simulink library "jud"  (Simulink 8.2)
settings: Solver=ode45  StartTime=0.0  StopTime=10.0  RelTol=1e-3
undefined symbols (not defined in the file or in its folder): ENUM_EPSADASABREASON_GEAR_POSITION_ERROR, ENUM_EPSADASABREASON_THERMAL_ERROR, ENUM_EPSADASABREASON_VEHICLE_SPEED_ERROR, ENUM_EPSLFCSTATUS_NOTAVAIL_PERM, ENUM_EPSLFCSTATUS_NOTAVAIL_TEMP, ENUM_EPSLFCSTATUS_OFF, ENUM_EPSLFCSTATUS_READY, ENUM_EPSLFCSTATUS_TRANSITION, ENUM_EPSLKASTATUS_NOTAVAIL_PERM, ENUM_EPSLKASTATUS_NOTAVAIL_TEMP, ENUM_EPSLKASTATUS_OFF, ENUM_EPSLKASTATUS_READY, ENUM_HMISTATE_ACTIVE, ENUM_KEYSWITCH_ON, ENUM_LFCSTATE_AUTOSTEERING, ENUM_LFCSTATE_STANDBY, ENUM_SENSORSTATE_NORMAL, FALSE, KAPP_VehicleWidth_m, KJUD_EPSLimition_kph, KJUD_EPSLimitionHysis_kph, KJUD_LFC4StandbyDelay_s, KJUD_SoftenTimerThr_s, TRUE, VJUD_LFCOffCount4LKAStandby_s, VJUD_LKAReActingDelay_s, VJUD_TLCTriggerReActingDelay_s
libraries: hcu_lib x12, simulink x10, jcc x1, jcw x1, jeb x1
(part 3 of 3)

== system jud/JUD/jud/JLKA/jka/LKA_LeftOperationalRecover_Conditions ==
  VIFO_LeftLaneCrossing_flg : Inport
  VPER_LaneC0L_m : Inport  Port=2
  VPER_LaneC1L_rad : Inport  Port=3
  Add1 : Sum  Inputs=+-
  C0L4Disabled : Constant  Value=-0.2
  C1L4Disabled : Constant  Value=-0.01
  C1L_Pos_sec : Constant  Value=0.5
  Compare To Zero : simulink/Logic and Bit Operations/Compare To Zero  relop=>=  OutDataTypeStr=boolean
  Gain2 : Gain  Gain=0.5
  "KAPP_VehicleWidth_m " : Constant  Value=KAPP_VehicleWidth_m
  Logical Operator4 : Logic  Inputs=3  AllPortsSameDT=off  OutDataTypeStr=boolean
  Logical Operator5 : Logic  Operator=OR  AllPortsSameDT=off  OutDataTypeStr=boolean
  Relational Operator4 : RelationalOperator  OutDataTypeStr=boolean
  Relational Operator5 : RelationalOperator  OutDataTypeStr=boolean
  Relational Operator6 : RelationalOperator  OutDataTypeStr=boolean
  Timer : hcu_lib/Timer  SystemSampleTime=-1
  VJUD_LKALeftOperationalRecover_flg : Outport
  wires:
  "KAPP_VehicleWidth_m "/1 -> Gain2/1
  Gain2/1 -> Add1/2
  VPER_LaneC0L_m/1 -> Add1/1
  VPER_LaneC1L_rad/1 -> Compare To Zero/1, Relational Operator4/1
  C1L4Disabled/1 -> Relational Operator4/2
  C0L4Disabled/1 -> Relational Operator5/2
  Add1/1 -> Relational Operator5/1  "VJUD_LaneC0L2Veh_m"
  Compare To Zero/1 -> Timer/Enable
  Timer/1 -> Relational Operator6/1
  C1L_Pos_sec/1 -> Relational Operator6/2
  Relational Operator4/1 -> Logical Operator4/1
  Relational Operator6/1 -> Logical Operator4/2
  Relational Operator5/1 -> Logical Operator4/3
  Logical Operator5/1 -> VJUD_LKALeftOperationalRecover_flg/1  "VJUD_LKALeftOperationalRecover_flg"
  Logical Operator4/1 -> Logical Operator5/1
  VIFO_LeftLaneCrossing_flg/1 -> Logical Operator5/2

== system jud/JUD/jud/JLKA/jka/LKA_NoADASFailre_Conditions ==
  VDHP_DisableLKA_flg : Inport
  Logical Operator1 : Logic  Operator=NOT  AllPortsSameDT=off  OutDataTypeStr=boolean
  VJUD_LKANoADASFailure_flg : Outport
  wires:
  Logical Operator1/1 -> VJUD_LKANoADASFailure_flg/1  "VJUD_LKANoADASFailure_flg"
  VDHP_DisableLKA_flg/1 -> Logical Operator1/1

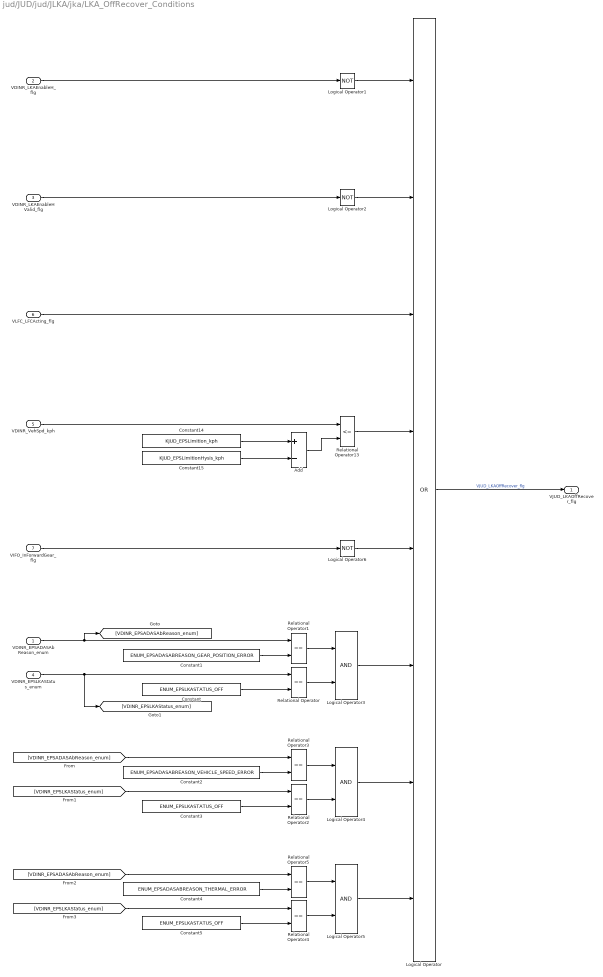
== system jud/JUD/jud/JLKA/jka/LKA_OffRecover_Conditions ==
  VDINR_EPSADASAbReason_enum : Inport
  VDINR_LKAEnableH_flg : Inport  Port=2
  VDINR_LKAEnableHValid_flg : Inport  Port=3
  VDINR_EPSLKAStatus_enum : Inport  Port=4
  VDINR_VehSpd_kph : Inport  Port=5
  VLFC_LFCActing_flg : Inport  Port=6
  VIFO_InForwardGear_flg : Inport  Port=7
  Add : Sum  Inputs=+-
  Constant : Constant  Value=ENUM_EPSLKASTATUS_OFF
  Constant1 : Constant  Value=ENUM_EPSADASABREASON_GEAR_POSITION_ERROR
  Constant14 : Constant  Value=KJUD_EPSLimition_kph
  Constant15 : Constant  Value=KJUD_EPSLimitionHysis_kph
  Constant2 : Constant  Value=ENUM_EPSADASABREASON_VEHICLE_SPEED_ERROR
  Constant3 : Constant  Value=ENUM_EPSLKASTATUS_OFF
  Constant4 : Constant  Value=ENUM_EPSADASABREASON_THERMAL_ERROR
  Constant5 : Constant  Value=ENUM_EPSLKASTATUS_OFF
  Logical Operator : Logic  Operator=OR  Inputs=8  AllPortsSameDT=off  OutDataTypeStr=boolean
  Logical Operator1 : Logic  Operator=NOT  AllPortsSameDT=off  OutDataTypeStr=boolean
  Logical Operator2 : Logic  Operator=NOT  AllPortsSameDT=off  OutDataTypeStr=boolean
  Logical Operator3 : Logic  AllPortsSameDT=off  OutDataTypeStr=boolean
  Logical Operator4 : Logic  AllPortsSameDT=off  OutDataTypeStr=boolean
  Logical Operator5 : Logic  AllPortsSameDT=off  OutDataTypeStr=boolean
  Logical Operator6 : Logic  Operator=NOT  AllPortsSameDT=off  OutDataTypeStr=boolean
  Relational Operator{,1..5} (6 alike) : RelationalOperator  Operator===  OutDataTypeStr=boolean
  Relational Operator13 : RelationalOperator  Operator=<=  OutDataTypeStr=boolean
  VJUD_LKAOffRecover_flg : Outport
  wires:
  Logical Operator/1 -> VJUD_LKAOffRecover_flg/1  "VJUD_LKAOffRecover_flg"
  Constant/1 -> Relational Operator/2
  VDINR_EPSLKAStatus_enum/1 -> [VDINR_EPSLKAStatus_enum], Relational Operator/1
  Relational Operator/1 -> Logical Operator3/2
  VDINR_EPSADASAbReason_enum/1 -> [VDINR_EPSADASAbReason_enum], Relational Operator1/1
  Constant1/1 -> Relational Operator1/2
  Relational Operator1/1 -> Logical Operator3/1
  [VDINR_EPSLKAStatus_enum] -> Relational Operator2/1
  Relational Operator2/1 -> Logical Operator4/2
  Constant2/1 -> Relational Operator3/2
  Relational Operator3/1 -> Logical Operator4/1
  [VDINR_EPSADASAbReason_enum] -> Relational Operator3/1
  Constant3/1 -> Relational Operator2/2
  [VDINR_EPSLKAStatus_enum] -> Relational Operator4/1
  Relational Operator4/1 -> Logical Operator5/2
  Constant4/1 -> Relational Operator5/2
  Relational Operator5/1 -> Logical Operator5/1
  [VDINR_EPSADASAbReason_enum] -> Relational Operator5/1
  Constant5/1 -> Relational Operator4/2
  VDINR_LKAEnableH_flg/1 -> Logical Operator1/1
  VDINR_LKAEnableHValid_flg/1 -> Logical Operator2/1
  VDINR_VehSpd_kph/1 -> Relational Operator13/1
  Constant14/1 -> Add/1
  Constant15/1 -> Add/2
  Add/1 -> Relational Operator13/2
  Logical Operator1/1 -> Logical Operator/1
  Logical Operator2/1 -> Logical Operator/2
  VLFC_LFCActing_flg/1 -> Logical Operator/3
  Relational Operator13/1 -> Logical Operator/4
  Logical Operator6/1 -> Logical Operator/5
  VIFO_InForwardGear_flg/1 -> Logical Operator6/1
  Logical Operator3/1 -> Logical Operator/6
  Logical Operator4/1 -> Logical Operator/7
  Logical Operator5/1 -> Logical Operator/8

== system jud/JUD/jud/JLKA/jka/LKA_Operational_Conditions ==
  VIFO_LeftLaneAvail_flg : Inport
  VIFO_RightLaneAvail_flg : Inport  Port=2
  VIFO_DriverTurningSignal_flg : Inport  Port=3
  VIFO_LKASpdInRange_flg : Inport  Port=4
  VIFO_Curvature4Disable_flg : Inport  Port=5
  VFCW_FCWStateHMI_enum : Inport  Port=6
  VAEB_AEBStateHMI_enum : Inport  Port=7
  Constant1 : Constant  Value=ENUM_HMISTATE_ACTIVE
  Constant2 : Constant  Value=ENUM_HMISTATE_ACTIVE
  Logical Operator : Logic  Inputs=6  AllPortsSameDT=off  OutDataTypeStr=boolean
  Logical Operator1 : Logic  Operator=OR  AllPortsSameDT=off  OutDataTypeStr=boolean
  Logical Operator2 : Logic  Operator=NOT  AllPortsSameDT=off  OutDataTypeStr=boolean
  Logical Operator3 : Logic  Operator=NOT  AllPortsSameDT=off  OutDataTypeStr=boolean
  Relational Operator2 : RelationalOperator  Operator=~=  OutDataTypeStr=boolean
  Relational Operator3 : RelationalOperator  Operator=~=  OutDataTypeStr=boolean
  VJUD_LKAOperationalReq_flg : Outport
  wires:
  Logical Operator/1 -> VJUD_LKAOperationalReq_flg/1  "VJUD_LKAOperationalReq_flg"
  VIFO_LeftLaneAvail_flg/1 -> Logical Operator1/1
  VIFO_RightLaneAvail_flg/1 -> Logical Operator1/2
  Logical Operator1/1 -> Logical Operator/1
  VIFO_DriverTurningSignal_flg/1 -> Logical Operator2/1
  VIFO_Curvature4Disable_flg/1 -> Logical Operator3/1
  VIFO_LKASpdInRange_flg/1 -> Logical Operator/2
  Logical Operator3/1 -> Logical Operator/3
  Logical Operator2/1 -> Logical Operator/4
  VFCW_FCWStateHMI_enum/1 -> Relational Operator2/1
  VAEB_AEBStateHMI_enum/1 -> Relational Operator3/1
  Constant1/1 -> Relational Operator2/2
  Constant2/1 -> Relational Operator3/2
  Relational Operator3/1 -> Logical Operator/6
  Relational Operator2/1 -> Logical Operator/5

== system jud/JUD/jud/JLKA/jka/LKA_RightAction_Conditions ==
  VDINR_EPSLKAStatus_enum : Inport
  VIFO_EPSStateChgAllow_flg : Inport  Port=2
  VIFO_TLCLTrigger_flg : Inport  Port=3
  VIFO_TLCRTrigger_flg : Inport  Port=4
  VLKA_LKAActing_flg : Inport  Port=5
  Constant1 : Constant  Value=ENUM_EPSLKASTATUS_READY
  Logical Operator : Logic  Operator=NOT  AllPortsSameDT=off  OutDataTypeStr=boolean
  Logical Operator3 : Logic  Inputs=5  AllPortsSameDT=off  OutDataTypeStr=boolean
  Logical Operator4 : Logic  Operator=NOT  AllPortsSameDT=off  OutDataTypeStr=boolean
  Relational Operator1 : RelationalOperator  RequirementInfo={} %GIDa_5d33ed69_386a_439d_af12_c65accea3bf3  Operator===  OutDataTypeStr=boolean
  Relational Operator2 : RelationalOperator  OutDataTypeStr=boolean
  Relational Operator3 : RelationalOperator  OutDataTypeStr=boolean
  Timer : hcu_lib/Timer  SystemSampleTime=-1
  Timer1 : hcu_lib/Timer  SystemSampleTime=-1
  VJUD_LKAReActingDelay_s : Constant  Value=VJUD_LKAReActingDelay_s
  VJUD_TLCTriggerReActingDelay_s : Constant  Value=VJUD_TLCTriggerReActingDelay_s
  VJUD_LKARightActionReq_flg : Outport
  wires:
  VIFO_TLCLTrigger_flg/1 -> Logical Operator/1
  Constant1/1 -> Relational Operator1/2
  VDINR_EPSLKAStatus_enum/1 -> Relational Operator1/1
  Logical Operator3/1 -> VJUD_LKARightActionReq_flg/1  "VJUD_LKARightActionReq_flg"
  VIFO_TLCRTrigger_flg/1 -> Logical Operator3/1
  Timer/1 -> Relational Operator2/1
  VJUD_LKAReActingDelay_s/1 -> Relational Operator2/2
  Logical Operator4/1 -> Timer/Enable
  VIFO_EPSStateChgAllow_flg/1 -> Logical Operator3/5
  Relational Operator1/1 -> Logical Operator3/4
  VLKA_LKAActing_flg/1 -> Logical Operator4/1
  Relational Operator2/1 -> Logical Operator3/2
  VJUD_TLCTriggerReActingDelay_s/1 -> Relational Operator3/2
  Relational Operator3/1 -> Logical Operator3/3
  Logical Operator/1 -> Timer1/Enable
  Timer1/1 -> Relational Operator3/1

== system jud/JUD/jud/JLKA/jka/LKA_RightOperationalRecover_Conditions ==
  VIFO_RightLaneCrossing_flg : Inport
  VPER_LaneC0R_m : Inport  Port=2
  VPER_LaneC1R_rad : Inport  Port=3
  Add1 : Sum
  C0R4Disabled : Constant  Value=0.2
  C1R4Disabled : Constant  Value=0.01
  C1R_nec_sec : Constant  Value=0.5
  Compare To Zero : simulink/Logic and Bit Operations/Compare To Zero  relop=<=  OutDataTypeStr=boolean
  Gain2 : Gain  Gain=0.5
  "KAPP_VehicleWidth_m " : Constant  Value=KAPP_VehicleWidth_m
  Logical Operator2 : Logic  Operator=OR  AllPortsSameDT=off  OutDataTypeStr=boolean
  Logical Operator4 : Logic  Inputs=3  AllPortsSameDT=off  OutDataTypeStr=boolean
  Relational Operator2 : RelationalOperator  Operator=<=  OutDataTypeStr=boolean
  Relational Operator3 : RelationalOperator  Operator=<=  OutDataTypeStr=boolean
  Relational Operator6 : RelationalOperator  OutDataTypeStr=boolean
  Timer : hcu_lib/Timer  SystemSampleTime=-1
  VJUD_LKARightOperationalRecover_flg : Outport
  wires:
  Add1/1 -> Relational Operator3/1  "VJUD_LaneC0R2Veh_m"
  "KAPP_VehicleWidth_m "/1 -> Gain2/1
  Gain2/1 -> Add1/2
  VPER_LaneC0R_m/1 -> Add1/1
  C1R4Disabled/1 -> Relational Operator2/2
  VPER_LaneC1R_rad/1 -> Compare To Zero/1, Relational Operator2/1
  Compare To Zero/1 -> Timer/Enable
  Timer/1 -> Relational Operator6/1
  C1R_nec_sec/1 -> Relational Operator6/2
  C0R4Disabled/1 -> Relational Operator3/2
  Relational Operator2/1 -> Logical Operator4/1
  Relational Operator6/1 -> Logical Operator4/2
  Logical Operator2/1 -> VJUD_LKARightOperationalRecover_flg/1  "VJUD_LKARightOperationalRecover_flg"
  Logical Operator4/1 -> Logical Operator2/1
  VIFO_RightLaneCrossing_flg/1 -> Logical Operator2/2
  Relational Operator3/1 -> Logical Operator4/3

== system jud/JUD/jud/JLKA/jka/LKA_StandbyRecover_Conditions ==
  VIFO_LaneNotAvail_flg : Inport
  VIFO_DriverTurningSignal_flg : Inport  Port=2
  VIFO_LKASpdInRange_flg : Inport  Port=3
  VIFO_Curvature4Disable_flg : Inport  Port=4
  VIFO_DriverStrFight_flg : Inport  Port=5
  VFCW_FCWStateHMI_enum : Inport  Port=6
  VAEB_AEBStateHMI_enum : Inport  Port=7
  Constant1 : Constant  Value=ENUM_HMISTATE_ACTIVE
  Constant2 : Constant  Value=ENUM_HMISTATE_ACTIVE
  Logical Operator : Logic  Operator=OR  Inputs=7  AllPortsSameDT=off  OutDataTypeStr=boolean
  Logical Operator1 : Logic  Operator=NOT  AllPortsSameDT=off  OutDataTypeStr=boolean
  Relational Operator2 : RelationalOperator  Operator===  OutDataTypeStr=boolean
  Relational Operator3 : RelationalOperator  Operator===  OutDataTypeStr=boolean
  VJUD_LKAStandbyRecover_flg : Outport
  wires:
  Logical Operator/1 -> VJUD_LKAStandbyRecover_flg/1  "VJUD_LKAStandbyRecover_flg"
  VIFO_DriverTurningSignal_flg/1 -> Logical Operator/2
  VIFO_LaneNotAvail_flg/1 -> Logical Operator/1
  VIFO_Curvature4Disable_flg/1 -> Logical Operator/4
  VIFO_DriverStrFight_flg/1 -> Logical Operator/5
  VIFO_LKASpdInRange_flg/1 -> Logical Operator1/1
  VFCW_FCWStateHMI_enum/1 -> Relational Operator2/1
  VAEB_AEBStateHMI_enum/1 -> Relational Operator3/1
  Constant1/1 -> Relational Operator2/2
  Constant2/1 -> Relational Operator3/2
  Relational Operator2/1 -> Logical Operator/6
  Relational Operator3/1 -> Logical Operator/7
  Logical Operator1/1 -> Logical Operator/3

== system jud/JUD/jud/JLKA/jka/LKA_TempFailureRecover_Conditions ==
  VDINR_EPSLKAStatus_enum : Inport
  VDHP_DisableADASFun_flg : Inport  Port=2
  Constant : Constant  Value=ENUM_EPSLKASTATUS_OFF
  Constant1 : Constant  Value=ENUM_EPSLKASTATUS_NOTAVAIL_PERM
  Logical Operator : Logic  Operator=OR  Inputs=3  AllPortsSameDT=off  OutDataTypeStr=boolean
  Relational Operator : RelationalOperator  Operator===  OutDataTypeStr=boolean
  Relational Operator2 : RelationalOperator  Operator===  OutDataTypeStr=boolean
  VJUD_LKATempFailureRecover_flg : Outport
  wires:
  Logical Operator/1 -> VJUD_LKATempFailureRecover_flg/1  "VJUD_LKATempFailureRecover_flg"
  VDHP_DisableADASFun_flg/1 -> Logical Operator/3
  Relational Operator/1 -> Logical Operator/1
  Constant/1 -> Relational Operator/2
  Relational Operator2/1 -> Logical Operator/2
  VDINR_EPSLKAStatus_enum/1 -> Relational Operator2/1, Relational Operator/1
  Constant1/1 -> Relational Operator2/2

== system jud/JUD/jud/JLKA/jka/LKA_Temporary_Conditions ==
  VDHP_DisableLKA_flg : Inport
  VDINR_EPSLKAStatus_enum : Inport  Port=2
  Constant : Constant  Value=ENUM_EPSLKASTATUS_NOTAVAIL_TEMP
  Logical Operator3 : Logic  Operator=OR  AllPortsSameDT=off  OutDataTypeStr=boolean
  Relational Operator : RelationalOperator  Operator===  OutDataTypeStr=boolean
  VJUD_LKATempFailureReq_flg : Outport
  wires:
  Constant/1 -> Relational Operator/2
  Logical Operator3/1 -> VJUD_LKATempFailureReq_flg/1  "VJUD_LKATempFailureReq_flg"
  VDINR_EPSLKAStatus_enum/1 -> Relational Operator/1
  VDHP_DisableLKA_flg/1 -> Logical Operator3/1
  Relational Operator/1 -> Logical Operator3/2
